simulink model "Cuk_Converter"  (R2022b)
settings: Solver=VariableStepAuto  StartTime=0.0  StopTime=0.1  RelTol=1e-3
libraries: spsSeriesRLCBranchLib x5, spsMeanLib x2, spsMultimeterLib x2, spsDiodeLib x1, spsMosfetLib x1, spsDCVoltageSourceLib x1, sps_lib x1
settings Model: Creator=Biplov Jha  LastModifiedBy=Biplov Jha

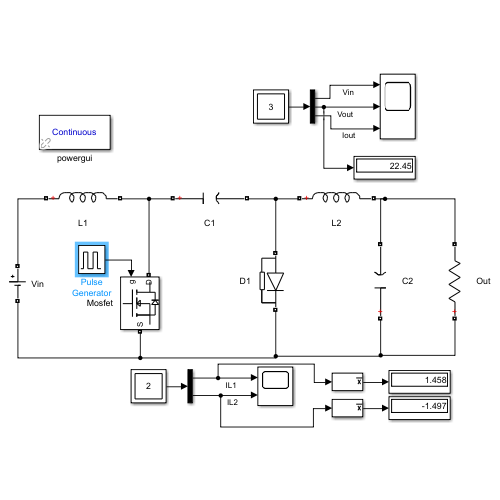
[thumbnail: Simulink's stored preview of the top-level diagram]
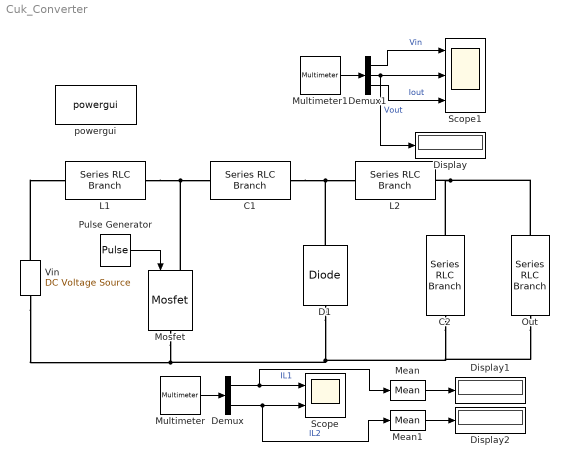
== system Cuk_Converter ==
  C1 : spsSeriesRLCBranchLib/Series RLC Branch  LConnTagsString=__new0  RConnTagsString=__new0  BranchType=C  Resistance=1  Inductance=1e-3  SetiL0=off  InitialCurrent=0  Capacitance=8e-6  Setx0=off  InitialVoltage=0  Measurements=None
  C2 : spsSeriesRLCBranchLib/Series RLC Branch  LConnTagsString=__new0  RConnTagsString=__new0  BranchType=C  Resistance=1  Inductance=1e-3  SetiL0=off  InitialCurrent=0  Capacitance=3.5e-6  Setx0=off  InitialVoltage=0  Measurements=None
  D1 : spsDiodeLib/Diode  Ron=0.001  Lon=0  Vf=0.8  IC=0  UseSnubber=0  Rs=500  Cs=250e-9  Measurements=off
  Demux : Demux  Outputs=2
  Demux1 : Demux  Outputs=3
  Display : Display
  Display1 : Display
  Display2 : Display
  L1 : spsSeriesRLCBranchLib/Series RLC Branch  LConnTagsString=__new0  RConnTagsString=__new0  BranchType=L  Resistance=1  Inductance=820e-6  SetiL0=off  InitialCurrent=0  Capacitance=1e-6  Setx0=off  InitialVoltage=0  Measurements=Branch current
  L2 : spsSeriesRLCBranchLib/Series RLC Branch  LConnTagsString=__new0  RConnTagsString=__new0  BranchType=L  Resistance=1  Inductance=681e-6  SetiL0=off  InitialCurrent=0  Capacitance=1e-6  Setx0=off  InitialVoltage=0  Measurements=Branch current
  Mean : spsMeanLib/Mean  Freq=60  Vinit=0  Ts=0
  Mean1 : spsMeanLib/Mean  Freq=60  Vinit=0  Ts=0
  "Mosfet " : spsMosfetLib/Mosfet  Ron=0.1  Lon=0  Rd=0.01  Vfd=0  IC=0  Rs=1e5  Cs=inf  Measurements=off
  Multimeter : spsMultimeterLib/Multimeter  L=5  sel=[3 4]  yselected={}  Gain=[1 1]  OutputType=Complex  PlotAtSimulationStop=off  PhasorSimulation=off
  Multimeter1 : spsMultimeterLib/Multimeter  L=5  sel=[2 1 5]  yselected={}  Gain=[1 1 1]  OutputType=Complex  PlotAtSimulationStop=off  PhasorSimulation=off
  Out : spsSeriesRLCBranchLib/Series RLC Branch  LConnTagsString=__new0  RConnTagsString=__new0  BranchType=R  Resistance=15  Inductance=1e-3  SetiL0=off  InitialCurrent=0  Capacitance=1e-6  Setx0=off  InitialVoltage=0  Measurements=Branch voltage and current
  Pulse Generator : DiscretePulseGenerator  PulseType=Time based  Period=1/(50e3)  PulseWidth=54.5
  Scope : Scope  NumInputPorts=2
  Scope1 : Scope  NumInputPorts=3
  Vin : spsDCVoltageSourceLib/DC Voltage Source  Amplitude=25  Measurements=Voltage
  powergui : sps_lib/powergui  Priority=1  SimulationMode=Continuous  SampleTime=50e-6  frequency=60  Iterations=50  frequencyindice=0  Pbase=100e6  ErrMax=1e-4  UnitsV=kV  UnitsW=MW  buscounter=0  FunctionMessages=off  echomessages=off  EnableUseOfTLC=off  CurrentSourceSwitches=off  DisableSnubberDevices=off  DisableRonSwitches=off  DisableVfSwitches=off  DisplayEquations=off  AutomaticDiscreteSolvers=off  SolverType=Tustin/Backward Euler (TBE)  Interpol=off  ExternalGateDelay=off  methode=off  Ts=100  x0status=blocks  SPID=on  SwTol=0  HookPort=off  NonlinearTolerance=1e-4  nMaxIteration=100  ContinueOnMaxIteration=off  RestoreLinks=warning  ResistiveCurrentMeasurement=off  Frange=[0:2:500]  Ylog=off  Xlog=on  ShowGrid=off  save=off  variable=ZData  structure=0  ZoomFFT=off  StartTime=0.0  cycles=1  DisplayStyle=1  fundamental=60  FreqAxis=off  MaxFrequency=1000  frequencyindicesteady=1  RmsSteady=1  display=off
  wires:
  Pulse Generator/1 -> "Mosfet "/1
  Multimeter/1 -> Demux/1
  Demux/1 -> Mean/1, Scope/1  "IL1"
  Demux/2 -> Mean1/1, Scope/2  "IL2"
  Demux1/2 -> Display/1, Scope1/2  "Vout"
  Demux1/1 -> Scope1/1  "Vin"
  Multimeter1/1 -> Demux1/1
  Demux1/3 -> Scope1/3  "Iout"
  Mean1/1 -> Display2/1
  Mean/1 -> Display1/1
  connections:
  Vin/RConn1 -- L1/LConn1
  L1/RConn1 -- C1/LConn1 -- "Mosfet "/LConn1
  C1/RConn1 -- L2/LConn1 -- D1/LConn1
  Vin/LConn1 -- Out/LConn1 -- C2/LConn1 -- D1/RConn1 -- "Mosfet "/RConn1
  Out/RConn1 -- C2/RConn1 -- L2/RConn1
